simulink model "chap04_02_33_mdl"  (R2013b)
settings: Solver=ode45  StartTime=0.0  StopTime=10.0  RelTol=1e-3
settings Model: Creator=Administrator  LastModifiedBy=sunzx.fnst

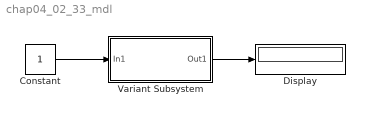
== system chap04_02_33_mdl ==
  Constant : Constant
  Display : Display
  Variant Subsystem : Subsystem  Variant=on  OverrideUsingVariant=Variant1
  wires:
  Constant/1 -> Variant Subsystem/1(In1)
  Variant Subsystem/1(Out1) -> Display/1

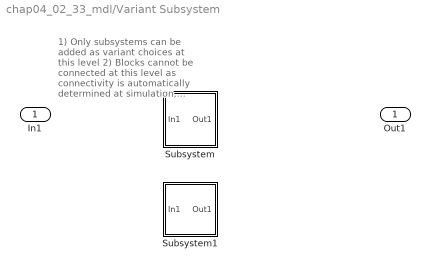
== system chap04_02_33_mdl/Variant Subsystem ==
  note: 1) Only subsystems can be added as variant choices at this level
      | 2) Blocks cannot be connected at this level as connectivity is
      | automatically determined at simulation, based on the active variant
  In1 : Inport
  Subsystem : Subsystem  VariantControl=Variant
  Subsystem1 : Subsystem  VariantControl=Variant1
  Out1 : Outport

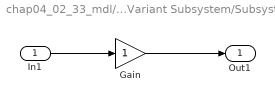
== system chap04_02_33_mdl/Variant Subsystem/Subsystem ==
  In1 : Inport
  Gain : Gain
  Out1 : Outport
  wires:
  In1/1 -> Gain/1
  Gain/1 -> Out1/1

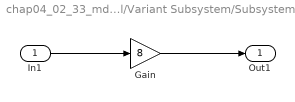
== system chap04_02_33_mdl/Variant Subsystem/Subsystem1 ==
  In1 : Inport
  Gain : Gain  Gain=8
  Out1 : Outport
  wires:
  In1/1 -> Gain/1
  Gain/1 -> Out1/1
